simulink model "IMUBaroModel"  (R2025b)
settings: Solver=VariableStepAuto  StartTime=0.0  StopTime=25  MaxStep=.05  RelTol=1e-3
StopFcn:
  | addpath("OutputData\");
  | 
  | processOutFile();
model workspace (MAT data in the model file):
  mass = 0.5
libraries: simulink x3, aerolibanim x1
settings Model: Creator=emmat  LastModifiedBy=emmat
settings DataIOCC: InspectSignalLogs=on  SignalLoggingName=logsoutput  OutputOption=SpecifiedOutputTimes  OutputTimes=[0:0.0025:17.8]

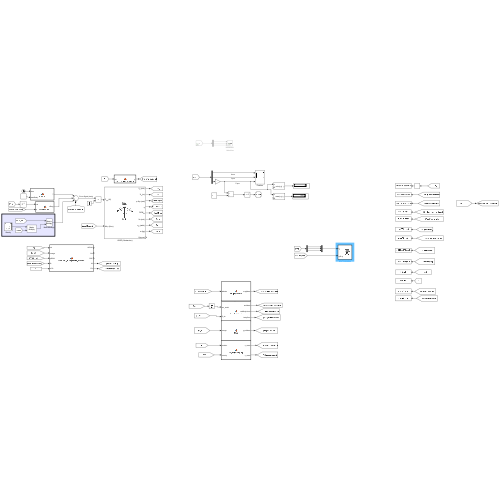
[thumbnail: Simulink's stored preview of the top-level diagram]
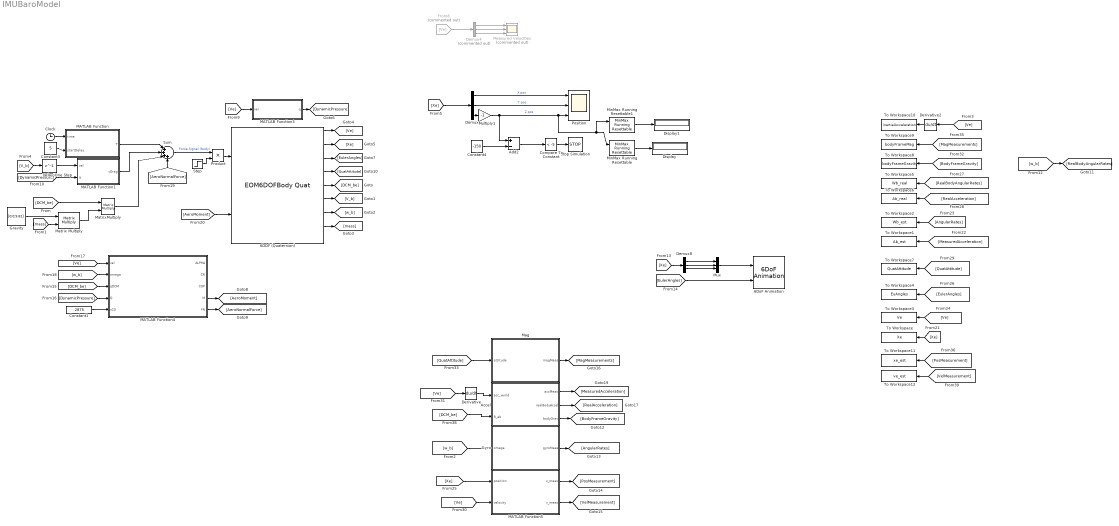
== system IMUBaroModel ==
  6DOF (Quaternion) : EOM6DOFBodyQuat  Vm_0=[.01 0 0]  eul_0=[deg2rad(0) deg2rad(85) deg2rad(0)]  mass_0=.44  inertia=[.009 0 0; 0 0.0152 0; 0 0 0.0152];  mass_flag=on
  6DoF Animation : aerolibanim/6DoF Animation  u1=[-100 100 -100 100 -200 250]  u2=0.1  u3=25  u4=[4000 0 -5000]  u5=Fixed position  u6=[0 200 100]  u7=50  u8=on
  Accel : MATLAB Function  TreatAsAtomicUnit=on  SystemSampleTime=1/400
      settings: AttributesFormatString=%<SystemSampleTime>
  Add2 : Sum  Inputs=+-
  Clock : Clock
  Compare To Constant : simulink/Logic and Bit Operations/Compare To Constant  relop=<  const=-5  OutDataTypeStr=boolean
  Constant1 : Constant  Value=.2875
  Constant3 : Constant  Value=5
  Constant4 : Constant  Value=-150
  Delay One Step : Delay  DelayLength=1
  Demux : Demux  Outputs=3
  Demux4 : Demux  Commented=on  Outputs=3
  Demux8 : Demux  Outputs=3
  Derivative : Derivative
  Derivative2 : Derivative
  Display : Display
  Display1 : Display
  From8 : From  Commented=on  GotoTag=Ve
  Gravity : Constant  Value=[0;0;9.81]  VectorParams1D=off
  Gyro : MATLAB Function  TreatAsAtomicUnit=on  SystemSampleTime=1/400
      settings: AttributesFormatString=%<SystemSampleTime>
  MATLAB Function : MATLAB Function  TreatAsAtomicUnit=on
  MATLAB Function1 : MATLAB Function  TreatAsAtomicUnit=on
  MATLAB Function3 : MATLAB Function  TreatAsAtomicUnit=on
  MATLAB Function4 : MATLAB Function  TreatAsAtomicUnit=on
  MATLAB Function5 : MATLAB Function  TreatAsAtomicUnit=on  SystemSampleTime=1/400
  Mag : MATLAB Function  TreatAsAtomicUnit=on  SystemSampleTime=1/400
      settings: AttributesFormatString=%<SystemSampleTime>
  Matrix Multiply : Product  Multiplication=Matrix(*)
  MatrixMultiply : Product  Multiplication=Matrix(*)
  Measured Velocities : Scope  Commented=on  NumInputPorts=3
      settings: ActiveDisplayYMinimum=-2.4223092485704854  ActiveDisplayYMaximum=13.491663232439137  DataLoggingVariableName=ScopeData5
  MinMax Running Resettable : simulink/Math Operations/MinMax Running Resettable  Function=max  vinit=0.0
  MinMax Running Resettable1 : simulink/Math Operations/MinMax Running Resettable  Function=min  vinit=0.0
  Multiply1 : Gain  Gain=-1
  Mux : Mux  Inputs=3
  Position : Scope  NumInputPorts=3
      settings: ActiveDisplayYMinimum=-1  ActiveDisplayYMaximum=1
  Product : Product
  Step : Step  Time=5  SampleTime=0
  Stop Simulation : Stop
  Sum : Sum  Inputs=|++++
  To Workspace : ToWorkspace  VariableName=Xe  SaveFormat=Timeseries  SampleTime=-1
  To Workspace1 : ToWorkspace  VariableName=Ab_est  SaveFormat=Timeseries  SampleTime=-1
  To Workspace10 : ToWorkspace  VariableName=inertialAcceleration  SaveFormat=Timeseries  SampleTime=-1
  To Workspace11 : ToWorkspace  VariableName=xe_est  SaveFormat=Timeseries  SampleTime=-1
  To Workspace12 : ToWorkspace  VariableName=ve_est  SaveFormat=Timeseries  SampleTime=-1
  To Workspace2 : ToWorkspace  VariableName=Wb_est  SaveFormat=Timeseries  SampleTime=-1
  To Workspace3 : ToWorkspace  VariableName=Ve  SaveFormat=Timeseries  SampleTime=-1
  To Workspace4 : ToWorkspace  VariableName=EuAngles  SaveFormat=Timeseries  SampleTime=-1
  To Workspace5 : ToWorkspace  VariableName=Wb_real  SaveFormat=Timeseries  SampleTime=-1
  To Workspace6 : ToWorkspace  VariableName=Ab_real  SaveFormat=Timeseries  SampleTime=-1
  To Workspace7 : ToWorkspace  VariableName=QuatAttitude  SaveFormat=Timeseries  SampleTime=-1
  To Workspace8 : ToWorkspace  VariableName=bodyFrameGravity  SaveFormat=Timeseries  SampleTime=-1
  To Workspace9 : ToWorkspace  VariableName=bodyFrameMag  SaveFormat=Timeseries  SampleTime=-1
  wires:
  6DOF (Quaternion)/5 -> [DCM_be]
  Clock/1 -> MATLAB Function/1(time)
  Sum/1 -> Product/1  "Force Signal (body)"
  Demux/3 -> Multiply1/1
  Demux/2 -> Position/2  "Y pos"
  Demux/1 -> Position/1  "X pos"
  [DCM_be] -> MatrixMultiply/1
  Matrix Multiply/1 -> MatrixMultiply/2
  MATLAB Function/1(T) -> Sum/1
  Multiply1/1 -> Add2/1, MinMax Running Resettable1/1, MinMax Running Resettable/1, Position/3  "Z pos"
  Compare To Constant/1 -> Stop Simulation/1
  6DOF (Quaternion)/6 -> [V_b]
  6DOF (Quaternion)/7 -> [w_b]
  6DOF (Quaternion)/8 -> [mass]
  Gravity/1 -> Matrix Multiply/1
  [mass] -> Matrix Multiply/2
  MatrixMultiply/1 -> Sum/3
  6DOF (Quaternion)/1 -> [Ve]
  [V_b] -> Delay One Step/1
  6DOF (Quaternion)/2 -> [Xe]
  [Xe] -> Demux/1
  MATLAB Function1/1(vDrag) -> Sum/2
  Delay One Step/1 -> MATLAB Function1/1(vel)
  MinMax Running Resettable/1 -> Display/1
  From8/1 -> Demux4/1
  Demux4/2 -> Measured Velocities/2
  Demux4/1 -> Measured Velocities/1
  Demux4/3 -> Measured Velocities/3
  [Ve] -> MATLAB Function3/1(vel)
  MATLAB Function3/1(q) -> [DynamicPressure]
  [DynamicPressure] -> MATLAB Function1/2(q)
  6DOF (Quaternion)/3 -> [EulerAngles]
  [Xe] -> Demux8/1
  [EulerAngles] -> 6DoF Animation/2
  Demux8/2 -> Mux/2
  Demux8/1 -> Mux/1
  Mux/1 -> 6DoF Animation/1
  Demux8/3 -> Mux/3
  [DCM_be] -> MATLAB Function4/3(qDCM)
  [DynamicPressure] -> MATLAB Function4/4(Q)
  Constant1/1 -> MATLAB Function4/5(xCG)
  MATLAB Function4/4(M) -> [AeroMoment]
  MATLAB Function4/5(FN) -> [AeroNormalForce]
  [w_b] -> MATLAB Function4/2(omega)
  [AeroMoment] -> 6DOF (Quaternion)/2
  [AeroNormalForce] -> Sum/4
  [Ve] -> MATLAB Function4/1(vel)
  6DOF (Quaternion)/4 -> [QuatAttitude]
  [Xe] -> To Workspace/1
  [MeasuredAcceleration] -> To Workspace1/1
  [AngularRates] -> To Workspace2/1
  [Ve] -> To Workspace3/1
  [EulerAngles] -> To Workspace4/1
  [RealBodyAngularRates] -> To Workspace5/1
  [RealAcceleration] -> To Workspace6/1
  [QuatAttitude] -> To Workspace7/1
  Constant3/1 -> MATLAB Function/2(startDelay)
  Step/1 -> Product/2
  Product/1 -> 6DOF (Quaternion)/1
  MinMax Running Resettable1/1 -> Display1/1
  [BodyFrameGravity] -> To Workspace8/1
  Mag/1(magMeas) -> [MagMeasurements]
  [QuatAttitude] -> Mag/1(attitude)
  [MagMeasurements] -> To Workspace9/1
  Accel/1(accMeas) -> [MeasuredAcceleration]
  [w_b] -> Gyro/1(omega)
  Gyro/1(gyroMeas) -> [AngularRates]
  [Ve] -> Derivative2/1
  Derivative2/1 -> To Workspace10/1
  [Ve] -> Derivative/1
  Derivative/1 -> Accel/1(acc_world)
  [DCM_be] -> Accel/2(R_eb)
  Add2/1 -> Compare To Constant/1
  Constant4/1 -> Add2/2
  [w_b] -> [RealBodyAngularRates]
  Accel/3(bodyGrav) -> [BodyFrameGravity]
  [Xe] -> MATLAB Function5/1(position)
  [Ve] -> MATLAB Function5/2(velocity)
  MATLAB Function5/1(x_meas) -> [PosMeasurement]
  MATLAB Function5/2(v_meas) -> [VelMeasurement]
  [PosMeasurement] -> To Workspace11/1
  [VelMeasurement] -> To Workspace12/1
  Accel/2(realBodyAccel) -> [RealAcceleration]

== matlab function IMUBaroModel/MATLAB Function1 ==
  data: vel input; vDrag output; q input
function vDrag = calculate_drag(vel, q)
    arguments
        vel (3,1)double % body velocity 
        q
    end

    reference_area  = 0.00283; % m^2
    drag_coeff      = 0.36; 
    
    vel_norm = norm(vel); 

    if vel_norm < 1e-6
        vDrag = [0;0;0];
        return
    end


    vDrag = -(vel/vel_norm) * drag_coeff * reference_area * q;

== matlab function IMUBaroModel/MATLAB Function ==
  data: T output; time input; startDelay input
% Returns thrust provided by motor provided in csv file
% This gives a thrust vector with thrust in the x body axis 
function T = tThrust(time, startDelay)
    arguments (Input)
        time double
        startDelay double
    end

    arguments(Output)
        T (3,1)double
    end
    
    persistent data
    persistent tTime 
    persistent tThrust

    if isempty(data)
        disp('Reading data...')
        
        data = load("C:\Users\emmat\Desktop\Year5\AERO626\Project\ThrustCurves\AeroTech_E24C.mat"); 

        tTime = data.tTime;
        tThrust = data.tThrust; 

    end

    if time-startDelay > tTime(end) || time < startDelay
        T = [0;0;0];
        return
    end

    thrust = interp1(tTime, tThrust, time-startDelay, 'linear'); 

    T = [thrust;0;0];

== matlab function IMUBaroModel/MATLAB Function3 ==
  data: vel input; q output
function q = calc_dynamic_pressure(vel)
    rho = 1.225; % kg/m^3
    q = 1/2 * rho * norm(vel)^2;

== matlab function IMUBaroModel/MATLAB Function4 ==
  data: vel input; omega input; ALPHA output; qDCM input; Q input; xCG input; CN output; COP output; M output; FN output
function [ALPHA, CN, COP, M, FN] = calculate_aerodynamic_moment(vel, omega, qDCM, Q, xCG)
    coder.varsize("aoa")
    coder.varsize("cop")
    coder.varsize("cna")

    persistent aoa cop cna 
    
    reference_area  = 0.00283; % m^2
    
    if isempty(aoa)
        data = load("C:\Users\emmat\Desktop\Year5\AERO626\Project\RocketData\vehicleData.mat");

        aoa = data.aoa;
        cop = data.cop;
        cna = data.cna;
    end

    norm_v = vel / norm(vel); 

    norm_pointing = qDCM'*[1;0;0];

    cosTheta = max(min(dot(norm_v, norm_pointing)/(norm(norm_v)*norm(norm_pointing)),1),-1); 
    ALPHA = acos(cosTheta); 

    CN  = interp1(aoa, cna, ALPHA,"linear") * ALPHA;
    COP = interp1(aoa, cop, ALPHA,"linear");
    
    % scalar normal force
    F = CN * Q * reference_area; 

    % lever arm in body frame
    R = [COP - xCG;0;0];

    % Projection of vel onto pointing
    proj_v_p = dot(norm_v, norm_pointing) * norm_pointing;

    % negative perpendicular component of velocity
    perp_V = -(proj_v_p-norm_v);

    % normal force vector 
    FN = qDCM * F * perp_V/norm(perp_V);

    if any(isnan(FN))
        FN = zeros(3,1);
    end
    
    % Damping moment
    cm_q = .08;
    
    M_damping = -cm_q * omega * Q * reference_area; 

    % Restoring moment in the world frame
    M = cross(R, FN) + M_damping;

== matlab function IMUBaroModel/Mag ==
  data: attitude input; magMeas output
function magMeas = Magnetometer(attitude)
    bias    = [0 0 0]';

    % NED Magnetic Magnitudes in microTesla
    NED     = [27.5550, -2.4169, -16.0849]';

    Pvv = diag([.01 .01 .01]);  

    noise   =  chol(Pvv, "lower")*randn(3,1);
    

    magMeas = quat2dcm(attitude')*NED + noise + bias;     
end

== matlab function IMUBaroModel/MATLAB Function5 ==
  data: position input; x_meas output; velocity input; v_meas output
function [x_meas,v_meas] = RayleighSampling(position, velocity)
    
    % Sigma defined by 2.5 50% CEP by NEO6M gps
    r_sigma = 1.177; 
   
    r = r_sigma * sqrt(-2*log(1-rand())); 

    theta = 2*pi*rand(); 

    dr = [r * cos(theta); r * sin(theta); 1.5*r_sigma*randn()] ;
    dv = [.1*randn(); .1*randn(); .2*randn()]; 
    
    x_meas = position + dr; 
    v_meas = velocity + dv; 
end

== matlab function IMUBaroModel/Accel ==
  data: acc_world input; accMeas output; realBodyAccel output; R_eb input; bodyGrav output
function [accMeas, realBodyAccel, bodyGrav]= Accelerometer(acc_world, R_eb)
    bias = [0;0;0];
    g_world = [0; 0; 9.81];

    f_body = R_eb * (acc_world - g_world);   % specific force in body frame
    
    realBodyAccel = f_body; 

    bodyGrav = R_eb * (-g_world); 

    Pvv  = diag([.017 .017 .017]);
    noise = chol(Pvv,"lower")*randn(3,1);

    accMeas = f_body + bias + noise;
end

== matlab function IMUBaroModel/Gyro ==
  data: omega input; gyroMeas output
function gyroMeas = Gyro(omega)

    bias    = [0 0 0]';

    Pvv     = diag([.0046 .0046 .0046]);  

    noise   =  chol(Pvv, "lower")*randn(3,1);
    
    gyroMeas = omega + noise + bias; 

end
